simulink model "compliant"  (R2023b)
settings: Solver=VariableStepAuto  StartTime=0.0  StopTime=50  RelTol=1e-3
settings Model: Creator=Rutvik  LastModifiedBy=bhara
settings ModelReferenceCC: EnableRefExpFcnMdlSchedulingChecks=on

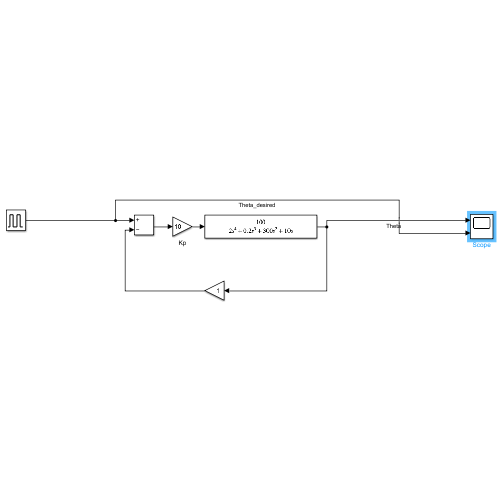
[thumbnail: Simulink's stored preview of the top-level diagram]
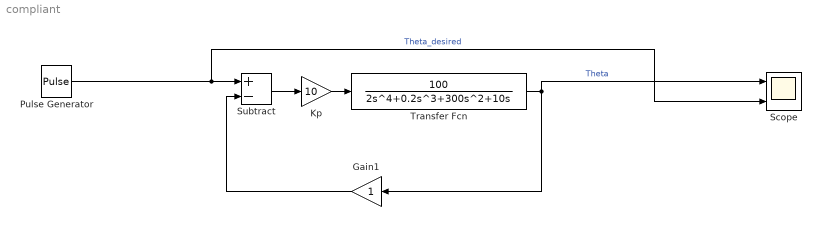
== system compliant ==
  Gain1 : Gain
  Kp : Gain  Gain=10
  Pulse Generator : DiscretePulseGenerator  PulseType=Time based  Period=5  PulseWidth=50
  Scope : Scope  NumInputPorts=2
  Subtract : Sum  Inputs=+-
  Transfer Fcn : TransferFcn  Numerator=[100]  Denominator=[2 0.2 300 10 0]
  wires:
  Kp/1 -> Transfer Fcn/1
  Transfer Fcn/1 -> Scope/1, Gain1/1  "Theta"
  Gain1/1 -> Subtract/2
  Pulse Generator/1 -> Scope/2, Subtract/1  "Theta_desired"
  Subtract/1 -> Kp/1
